simulink model "CSC"  (R2022a)
settings: Solver=VariableStepAuto  StartTime=0.0  StopTime=0.1  RelTol=1e-3
undefined symbols (not defined in the file): gray, Rec, SDTV
libraries: hdlsllib x16, visionhdlio x4, visionhdlconversions x2, dspvision x2
settings Model: Creator=HACKone  LastModifiedBy=HACKone

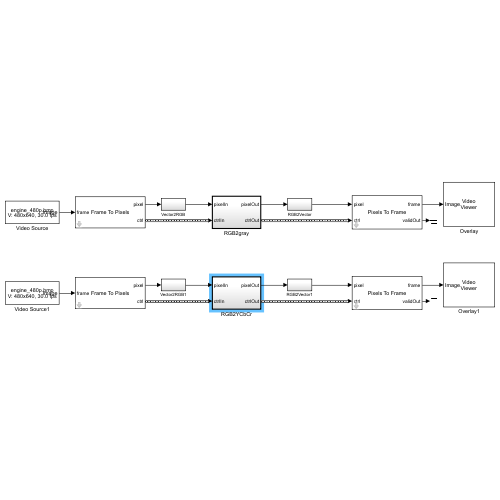
[thumbnail: Simulink's stored preview of the top-level diagram]
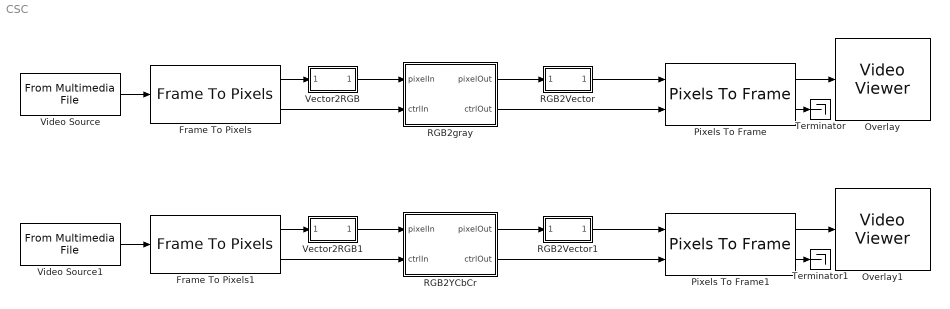
== system CSC ==
  Frame To Pixels : visionhdlio/Frame To Pixels  NumComponents=3  NumPixels=1  VideoFormat=480p  ActivePixelsPerLine=640  ActiveVideoLines=480  TotalPixelsPerLine=800  TotalVideoLines=525  StartingActiveLine=36  FrontPorch=16  SampleTime=0  VideoFormatCache=480p  ActivePixelsPerLineCache=32  ActiveVideoLinesCache=18  TotalPixelsPerLineCache=42  TotalVideoLinesCache=28  StartingActiveLineCache=6  FrontPorchCache=5
      settings: SourceProductBaseCode=VT
  Frame To Pixels1 : visionhdlio/Frame To Pixels  NumComponents=3  NumPixels=1  VideoFormat=480p  ActivePixelsPerLine=640  ActiveVideoLines=480  TotalPixelsPerLine=800  TotalVideoLines=525  StartingActiveLine=36  FrontPorch=16  SampleTime=0  VideoFormatCache=480p  ActivePixelsPerLineCache=32  ActiveVideoLinesCache=18  TotalPixelsPerLineCache=42  TotalVideoLinesCache=28  StartingActiveLineCache=6  FrontPorchCache=5
      settings: SourceProductBaseCode=VT
  Overlay : VideoViewer  colormapValue=gray(256)  FigPos=[435 527 354 280]
  Overlay1 : VideoViewer  colormapValue=gray(256)  FigPos=[843 539 354 280]
  Pixels To Frame : visionhdlio/Pixels To Frame  NumComponents=3  NumPixels=1  VideoFormat=480p  ActivePixelsPerLine=640  ActiveVideoLines=480  TotalPixelsPerLine=800  TotalVideoLines=525  VideoFormatCache=480p  ActivePixelsPerLineCache=32  ActiveVideoLinesCache=18  TotalPixelsPerLineCache=42  TotalVideoLinesCache=28
      settings: SourceProductBaseCode=VT
  Pixels To Frame1 : visionhdlio/Pixels To Frame  NumComponents=3  NumPixels=1  VideoFormat=480p  ActivePixelsPerLine=640  ActiveVideoLines=480  TotalPixelsPerLine=800  TotalVideoLines=525  VideoFormatCache=480p  ActivePixelsPerLineCache=32  ActiveVideoLinesCache=18  TotalPixelsPerLineCache=42  TotalVideoLinesCache=28
      settings: SourceProductBaseCode=VT
  RGB2Vector : Subsystem
  RGB2Vector1 : Subsystem
  RGB2YCbCr : Subsystem  TreatAsAtomicUnit=on
  RGB2gray : Subsystem  TreatAsAtomicUnit=on
  Terminator : Terminator
  Terminator1 : Terminator
  Vector2RGB : Subsystem
  Vector2RGB1 : Subsystem
  Video Source : dspvision/From Multimedia File  inputFilename=D:\datasets\test_images\engine_480p.bmp  readRange=[1 Inf]  loop=on  numPlays=inf  outputStreams=Video only  videoDataType=uint8  audioDataType=int16  inheritSampleTime=off  userDefinedSampleTime=1/30  noAudioOutput=off  isIntensityVideo=off  fourcc=RGB  colorVideoFormat=One multidimensional signal  outputEOF=off  dataOrg=Column-major  audioFrameSize=1024  computeAudioFrameSize=off  outSamplingMode=Sample based
  Video Source1 : dspvision/From Multimedia File  inputFilename=D:\datasets\test_images\engine_480p.bmp  readRange=[1 Inf]  loop=on  numPlays=inf  outputStreams=Video only  videoDataType=uint8  audioDataType=int16  inheritSampleTime=off  userDefinedSampleTime=1/30  noAudioOutput=off  isIntensityVideo=off  fourcc=RGB  colorVideoFormat=One multidimensional signal  outputEOF=off  dataOrg=Column-major  audioFrameSize=1024  computeAudioFrameSize=off  outSamplingMode=Sample based
  wires:
  RGB2gray/2(ctrlOut) -> Pixels To Frame/2
  RGB2gray/1(pixelOut) -> RGB2Vector/1(RGB)
  Frame To Pixels/1 -> Vector2RGB/1(RGBVector)
  Video Source/1 -> Frame To Pixels/1
  Pixels To Frame/2 -> Terminator/1
  Frame To Pixels/2 -> RGB2gray/2(ctrlIn)
  Pixels To Frame/1 -> Overlay/1
  Vector2RGB/1(RGB) -> RGB2gray/1(pixelIn)
  RGB2Vector/1(RGBVector) -> Pixels To Frame/1
  Frame To Pixels1/1 -> Vector2RGB1/1(RGBVector)
  RGB2Vector1/1(RGBVector) -> Pixels To Frame1/1
  Pixels To Frame1/1 -> Overlay1/1
  RGB2YCbCr/2(ctrlOut) -> Pixels To Frame1/2
  Frame To Pixels1/2 -> RGB2YCbCr/2(ctrlIn)
  RGB2YCbCr/1(pixelOut) -> RGB2Vector1/1(RGB)
  Video Source1/1 -> Frame To Pixels1/1
  Vector2RGB1/1(RGB) -> RGB2YCbCr/1(pixelIn)
  Pixels To Frame1/2 -> Terminator1/1

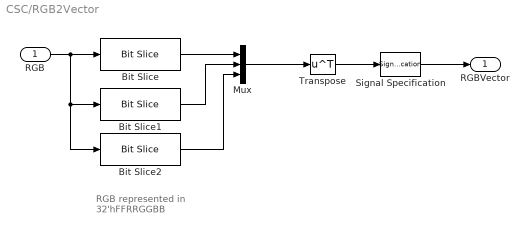
== system CSC/RGB2Vector ==
  note: RGB represented in
      | 32'hFFRRGGBB
  RGB : Inport
  Bit Slice : hdlsllib/Logic and Bit Operations/Bit Slice  lidx=23  ridx=16
  Bit Slice1 : hdlsllib/Logic and Bit Operations/Bit Slice  lidx=15  ridx=8
  Bit Slice2 : hdlsllib/Logic and Bit Operations/Bit Slice  lidx=7  ridx=0
  Mux : Mux  Inputs=3
  Signal Specification : SignalSpecification
  Transpose : Math  Operator=transpose  SignedPower=on
  RGBVector : Outport  VectorParamsAs1DForOutWhenUnconnected=off
  wires:
  Mux/1 -> Transpose/1
  Bit Slice/1 -> Mux/1
  Bit Slice2/1 -> Mux/3
  Bit Slice1/1 -> Mux/2
  RGB/1 -> Bit Slice2/1, Bit Slice1/1, Bit Slice/1
  Transpose/1 -> Signal Specification/1
  Signal Specification/1 -> RGBVector/1

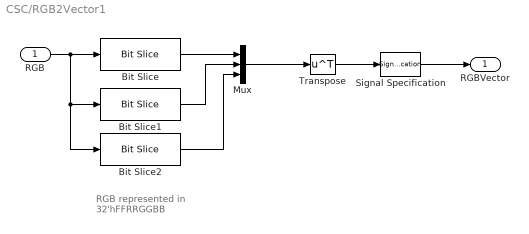
== system CSC/RGB2Vector1 ==
  note: RGB represented in
      | 32'hFFRRGGBB
  RGB : Inport
  Bit Slice : hdlsllib/Logic and Bit Operations/Bit Slice  lidx=23  ridx=16
  Bit Slice1 : hdlsllib/Logic and Bit Operations/Bit Slice  lidx=15  ridx=8
  Bit Slice2 : hdlsllib/Logic and Bit Operations/Bit Slice  lidx=7  ridx=0
  Mux : Mux  Inputs=3
  Signal Specification : SignalSpecification
  Transpose : Math  Operator=transpose  SignedPower=on
  RGBVector : Outport  VectorParamsAs1DForOutWhenUnconnected=off
  wires:
  Mux/1 -> Transpose/1
  Bit Slice/1 -> Mux/1
  Bit Slice2/1 -> Mux/3
  Bit Slice1/1 -> Mux/2
  RGB/1 -> Bit Slice2/1, Bit Slice1/1, Bit Slice/1
  Transpose/1 -> Signal Specification/1
  Signal Specification/1 -> RGBVector/1

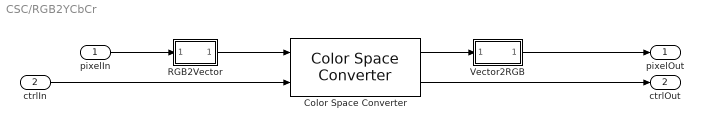
== system CSC/RGB2YCbCr ==
  pixelIn : Inport
  ctrlIn : Inport  Port=2
  Color Space Converter : visionhdlconversions/Color Space Converter  Conversion=RGB to YCbCr  ConversionStandard=Rec. 601 (SDTV)  ScanningStandard=1250/50/2:1  SimulateUsing=Code generation
      settings: SourceProductBaseCode=VT
  RGB2Vector : Subsystem
  Vector2RGB : Subsystem
  pixelOut : Outport  VectorParamsAs1DForOutWhenUnconnected=off
  ctrlOut : Outport  Port=2  VectorParamsAs1DForOutWhenUnconnected=off
  wires:
  ctrlIn/1 -> Color Space Converter/2
  pixelIn/1 -> RGB2Vector/1(RGB)
  Color Space Converter/2 -> ctrlOut/1
  Color Space Converter/1 -> Vector2RGB/1(RGBVector)
  RGB2Vector/1(RGBVector) -> Color Space Converter/1
  Vector2RGB/1(RGB) -> pixelOut/1

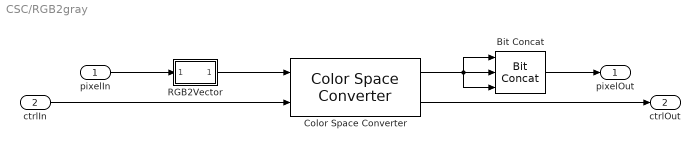
== system CSC/RGB2gray ==
  pixelIn : Inport
  ctrlIn : Inport  Port=2
  Bit Concat : hdlsllib/Logic and Bit Operations/Bit Concat  numInputs=3
      settings: SourceProductBaseCode=HD
  Color Space Converter : visionhdlconversions/Color Space Converter  Conversion=RGB to intensity  ConversionStandard=Rec. 601 (SDTV)  ScanningStandard=1250/50/2:1  SimulateUsing=Code generation
      settings: SourceProductBaseCode=VT
  RGB2Vector : Subsystem
  pixelOut : Outport  VectorParamsAs1DForOutWhenUnconnected=off
  ctrlOut : Outport  Port=2  VectorParamsAs1DForOutWhenUnconnected=off
  wires:
  ctrlIn/1 -> Color Space Converter/2
  pixelIn/1 -> RGB2Vector/1(RGB)
  Color Space Converter/2 -> ctrlOut/1
  Color Space Converter/1 -> Bit Concat/3, Bit Concat/2, Bit Concat/1
  RGB2Vector/1(RGBVector) -> Color Space Converter/1
  Bit Concat/1 -> pixelOut/1

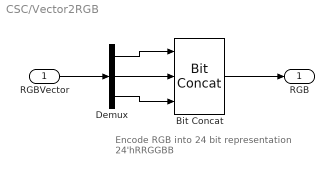
== system CSC/Vector2RGB ==
  note: Encode RGB into 24 bit representation
      | 24'hRRGGBB
  RGBVector : Inport
  Bit Concat : hdlsllib/Logic and Bit Operations/Bit Concat  numInputs=3
      settings: SourceProductBaseCode=HD
  Demux : Demux  Outputs=3
  RGB : Outport  VectorParamsAs1DForOutWhenUnconnected=off
  wires:
  Bit Concat/1 -> RGB/1
  RGBVector/1 -> Demux/1
  Demux/1 -> Bit Concat/1
  Demux/2 -> Bit Concat/2
  Demux/3 -> Bit Concat/3

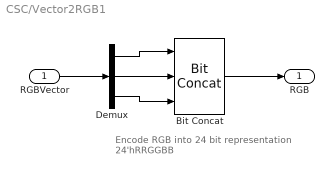
== system CSC/Vector2RGB1 ==
  note: Encode RGB into 24 bit representation
      | 24'hRRGGBB
  RGBVector : Inport
  Bit Concat : hdlsllib/Logic and Bit Operations/Bit Concat  numInputs=3
      settings: SourceProductBaseCode=HD
  Demux : Demux  Outputs=3
  RGB : Outport  VectorParamsAs1DForOutWhenUnconnected=off
  wires:
  Bit Concat/1 -> RGB/1
  RGBVector/1 -> Demux/1
  Demux/1 -> Bit Concat/1
  Demux/2 -> Bit Concat/2
  Demux/3 -> Bit Concat/3

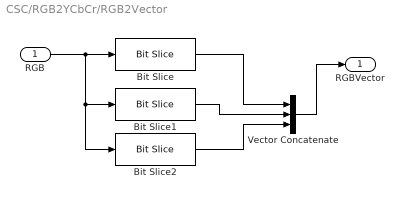
== system CSC/RGB2YCbCr/RGB2Vector ==
  RGB : Inport
  Bit Slice : hdlsllib/Logic and Bit Operations/Bit Slice  lidx=23  ridx=16
  Bit Slice1 : hdlsllib/Logic and Bit Operations/Bit Slice  lidx=15  ridx=8
  Bit Slice2 : hdlsllib/Logic and Bit Operations/Bit Slice  lidx=7  ridx=0
  Vector Concatenate : Concatenate  NumInputs=3  Mode=Multidimensional array  ConcatenateDimension=2
  RGBVector : Outport  VectorParamsAs1DForOutWhenUnconnected=off
  wires:
  RGB/1 -> Bit Slice2/1, Bit Slice1/1, Bit Slice/1
  Bit Slice/1 -> Vector Concatenate/1
  Bit Slice1/1 -> Vector Concatenate/2
  Bit Slice2/1 -> Vector Concatenate/3
  Vector Concatenate/1 -> RGBVector/1

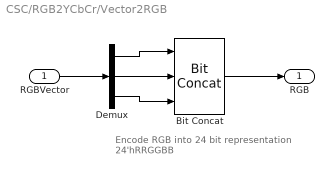
== system CSC/RGB2YCbCr/Vector2RGB ==
  note: Encode RGB into 24 bit representation
      | 24'hRRGGBB
  RGBVector : Inport
  Bit Concat : hdlsllib/Logic and Bit Operations/Bit Concat  numInputs=3
      settings: SourceProductBaseCode=HD
  Demux : Demux  Outputs=3
  RGB : Outport  VectorParamsAs1DForOutWhenUnconnected=off
  wires:
  Bit Concat/1 -> RGB/1
  RGBVector/1 -> Demux/1
  Demux/1 -> Bit Concat/1
  Demux/2 -> Bit Concat/2
  Demux/3 -> Bit Concat/3

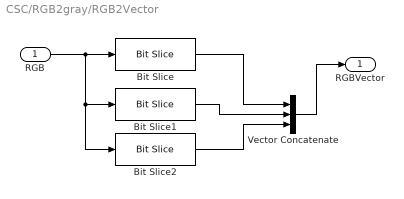
== system CSC/RGB2gray/RGB2Vector ==
  RGB : Inport
  Bit Slice : hdlsllib/Logic and Bit Operations/Bit Slice  lidx=23  ridx=16
  Bit Slice1 : hdlsllib/Logic and Bit Operations/Bit Slice  lidx=15  ridx=8
  Bit Slice2 : hdlsllib/Logic and Bit Operations/Bit Slice  lidx=7  ridx=0
  Vector Concatenate : Concatenate  NumInputs=3  Mode=Multidimensional array  ConcatenateDimension=2
  RGBVector : Outport  VectorParamsAs1DForOutWhenUnconnected=off
  wires:
  RGB/1 -> Bit Slice2/1, Bit Slice1/1, Bit Slice/1
  Bit Slice/1 -> Vector Concatenate/1
  Bit Slice1/1 -> Vector Concatenate/2
  Bit Slice2/1 -> Vector Concatenate/3
  Vector Concatenate/1 -> RGBVector/1
